simulink model "lab_8"  (R2020a)
settings: Solver=FixedStepAuto  StartTime=0.0  StopTime=20  FixedStep=0.01  RelTol=1e-3
undefined symbols (not defined in the file or in its folder): k_1, k_2, y_r
settings Model: Creator=bruno  LastModifiedBy=bruno

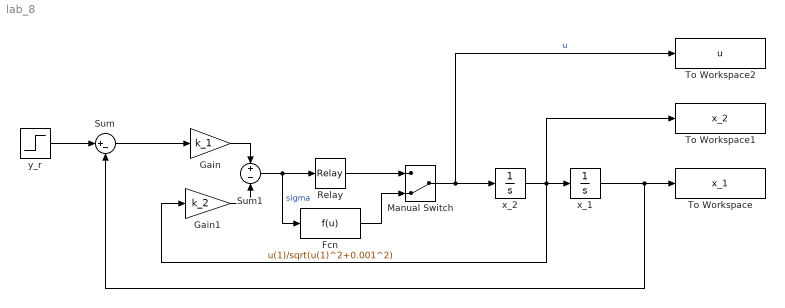
== system lab_8 ==
  Fcn : Fcn  Expr=u(1)/sqrt(u(1)^2+0.001^2)
  Gain : Gain  Gain=k_1
  Gain1 : Gain  Gain=k_2
  Manual Switch : ManualSwitch  CurrentSetting=0
  Relay : Relay  OnSwitchValue=0.2  OffSwitchValue=-0.2  OffOutputValue=-1
  Sum : Sum  Inputs=|+-
  Sum1 : Sum  Inputs=+|-
  To Workspace : ToWorkspace  VariableName=x_1  SaveFormat=Timeseries  SampleTime=-1
  To Workspace1 : ToWorkspace  VariableName=x_2  SaveFormat=Timeseries  SampleTime=-1
  To Workspace2 : ToWorkspace  VariableName=u  SaveFormat=Timeseries  SampleTime=-1
  x_1 : Integrator
  x_2 : Integrator
  y_r : Step  Time=2  After=y_r  SampleTime=0
  wires:
  x_2/1 -> Gain1/1, To Workspace1/1, x_1/1
  Manual Switch/1 -> To Workspace2/1, x_2/1  "u"
  y_r/1 -> Sum/1
  x_1/1 -> To Workspace/1, Sum/2
  Sum/1 -> Gain/1
  Sum1/1 -> Fcn/1, Relay/1  "sigma"
  Gain/1 -> Sum1/1
  Gain1/1 -> Sum1/2
  Fcn/1 -> Manual Switch/2
  Relay/1 -> Manual Switch/1
